simulink model "SimulinkODEexample"  (R2017b)
settings: Solver=FixedStepAuto  StartTime=0.0  StopTime=3.0  FixedStep=1  RelTol=1e-3
settings Model: Creator=toni  LastModifiedBy=toni

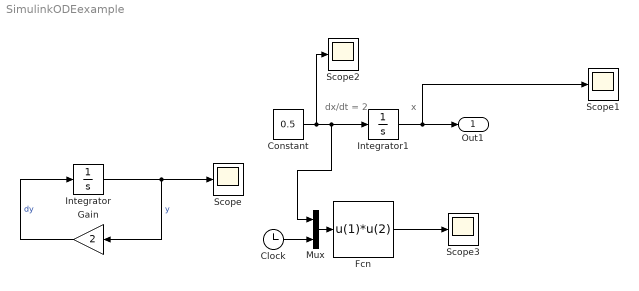
== system SimulinkODEexample ==
  note: x
  note: dx/dt = 2
  Clock : Clock
  Constant : Constant  Value=0.5
  Fcn : Fcn  Expr=u(1)*u(2)
  Gain : Gain  Gain=2
  Integrator : Integrator  InitialCondition=1
  Integrator1 : Integrator
  Mux : Mux  Inputs=2
  Scope{,1..3} (4 alike) : Scope
  Out1 : Outport
  wires:
  Integrator/1 -> Scope/1, Gain/1  "y"
  Gain/1 -> Integrator/1  "dy"
  Constant/1 -> Scope2/1, Mux/1, Integrator1/1
  Integrator1/1 -> Scope1/1, Out1/1
  Fcn/1 -> Scope3/1
  Mux/1 -> Fcn/1
  Clock/1 -> Mux/2
